simulink model "cbf_with_lead_accel_est"  (R2021a)
settings: Solver=FixedStepAuto  StartTime=0.0  StopTime=inf  FixedStep=0.05  RelTol=1e-3
undefined symbols (not defined in the file): Angular, Linear
libraries: robotlib x18
settings Model: Creator=ivory  LastModifiedBy=vanderbilt
settings SolverCC: AlgebraicLoopSolver=TrustRegion
settings OptimizationCC: EnhancedBackFolding=on  PassReuseOutputArgsAs=Individual arguments  ZeroExternalMemoryAtStartup=off  ZeroInternalMemoryAtStartup=off  MaxStackSize=64  OptimizeBlockOrder=speed  DifferentSizesBufferReuse=on  OptimizationCustomize=off  EfficientTunableParamExpr=on
settings DebuggingCC: ParameterTunabilityLossMsg=error  SFMachineParentedDataDiag=warning
settings HardwareCC: ProdBitPerPointer=32  ProdBitPerSizeT=32  ProdBitPerPtrDiffT=32  ProdLargestAtomicFloat=None  ProdIntDivRoundTo=Undefined  ProdEndianess=Unspecified  ProdWordSize=32  ProdHWDeviceType=Generic->Unspecified (assume 32-bit Generic)
settings SFSimCC: MATLABDynamicMemAlloc=off  SimTargetLang=C++
settings RTWCC: SystemTargetFile=ert.tlc  HardwareBoard=Robot Operating System (ROS)  TLCOptions="-aInlineSetEventsForThisBaseRateFcn=TLC_FALSE -aSuppressMultiTaskScheduler=TLC_FALSE  -aRateBasedStepFcn=0"  TemplateMakefile=ert_default_tmf  GenerateReport=on  Toolchain=Catkin  IncludeHyperlinkInReport=on  LaunchReport=on  TargetLang=C++  GenerateTraceInfo=on  GenerateTraceReport=on  GenerateTraceReportSl=on  GenerateTraceReportSf=on  GenerateTraceReportEml=on
settings CodeAppCC: ForceParamTrailComments=on  IgnoreCustomStorageClasses=off  OperatorAnnotations=on  SimulinkDataObjDesc=on  SFDataObjDesc=on  InsertBlockDesc=on
settings ERTTargetCC: SupportContinuousTime=on  SupportVariableSizeSignals=on

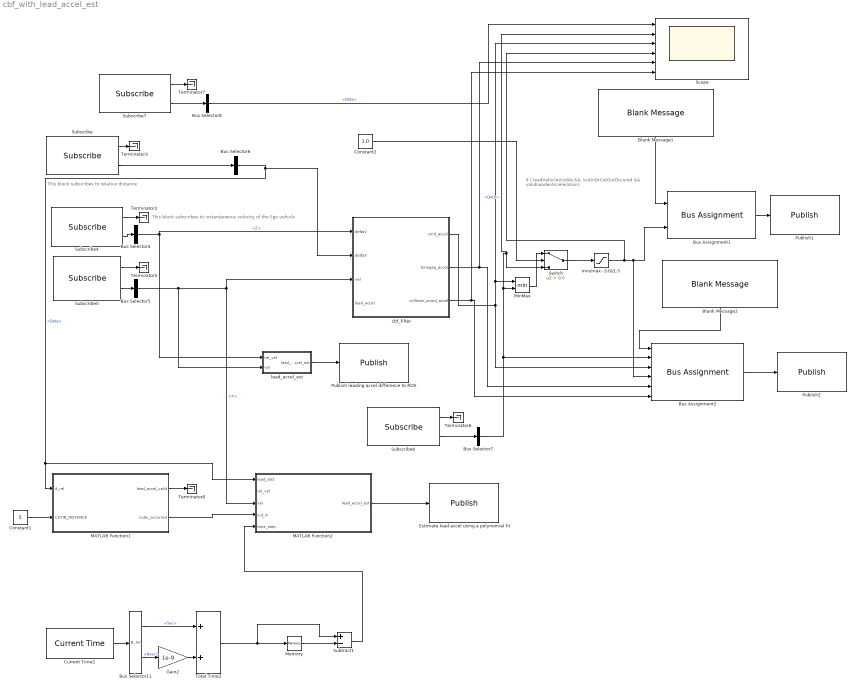
== system cbf_with_lead_accel_est ==
  note: if ( leadVehicleVisible && !cutInOrCutOutOccured && validLeaderAcceleration)
  note: This block subscribes
      | to relative distance
  note: This block subscribes to
      | instantaneous velocity of the Ego vehicle
  Blank Message1 : robotlib/Blank Message  messageClass=Message  entityType=std_msgs/Float64  messageType=std_msgs/Float64  SampleTime=inf  legacyBusStruct=off
  Blank Message2 : robotlib/Blank Message  messageClass=Message  entityType=geometry_msgs/Twist  messageType=geometry_msgs/Twist  SampleTime=inf  legacyBusStruct=off
  Bus Assignment1 : BusAssignment  AssignedSignals=Data
  Bus Assignment2 : BusAssignment  AssignedSignals=Linear.X,Linear.Y,Linear.Z,Angular.Y,Angular.Z
  Bus Selector11 : BusSelector  OutputSignals=Sec,Nsec
  Bus Selector4 : BusSelector  OutputSignals=Linear.Z
  Bus Selector5 : BusSelector  OutputSignals=Linear.X
  Bus Selector6 : BusSelector  OutputSignals=Data
  Bus Selector7 : BusSelector  OutputSignals=Data
  Bus Selector8 : BusSelector  OutputSignals=Data
  Constant1 : Constant  Value=5
  Constant2 : Constant  Value=1.0
  Current Time2 : robotlib/Current Time  OutputFormat=bus  SampleTime=-1  ModelName=micromodel
      settings: SourceProductBaseCode=RR
  Estimate lead accel using a polynomial fit : robotlib/Publish  topicSource=Specify your own  topic=/lead_accel_est/polynomial_est  messageType=std_msgs/Float64  legacyBusStruct=off  messageQueueLength=1
  Gain2 : Gain  Gain=1e-9
  MATLAB Function1 : MATLAB Function  TreatAsAtomicUnit=on
  MATLAB Function2 : MATLAB Function  TreatAsAtomicUnit=on
  Memory : Memory
  MinMax : MinMax  Inputs=2
  Publish leading accel difference to ROS : robotlib/Publish  topicSource=Specify your own  topic=/lead_accel_est/finite_diff  messageType=std_msgs/Float64  legacyBusStruct=off  messageQueueLength=1
  Publish1 : robotlib/Publish  topicSource=Specify your own  topic=cmd_accel  messageType=std_msgs/Float64  legacyBusStruct=off  messageQueueLength=1
  Publish2 : robotlib/Publish  topicSource=Specify your own  topic=/cbf/cbf_debug  messageType=geometry_msgs/Twist  legacyBusStruct=off  messageQueueLength=1
  Scope : Scope  NumInputPorts=6
  Subscribe : robotlib/Subscribe  topicSource=Specify your own  topic=lead_dist  messageType=std_msgs/Float64  SampleTime=-1  legacyBusStruct=off  messageQueueLength=1
  Subscribe4 : robotlib/Subscribe  topicSource=Specify your own  topic=rel_vel  messageType=geometry_msgs/Twist  SampleTime=-1  legacyBusStruct=off  messageQueueLength=1
  Subscribe5 : robotlib/Subscribe  topicSource=Specify your own  topic=vel  messageType=geometry_msgs/Twist  SampleTime=-1  legacyBusStruct=off  messageQueueLength=1
  Subscribe6 : robotlib/Subscribe  topicSource=Specify your own  topic=cmd_accel_pre  messageType=std_msgs/Float64  SampleTime=-1  legacyBusStruct=off  messageQueueLength=1
  Subscribe7 : robotlib/Subscribe  topicSource=Specify your own  topic=/car/hud/mini_car_enable  messageType=std_msgs/Bool  SampleTime=-1  legacyBusStruct=off  messageQueueLength=1
  Subtract1 : Sum  Inputs=+-
  Switch : Switch  Criteria=u2 > Threshold  Threshold=0.5
  Terminator{2..3,5..8} (6 alike) : Terminator
  Total Time2 : Sum
  cbf_filter : Subsystem
  lead_accel_est : Subsystem
  min/max -3.0//1.5 : Saturate  UpperLimit=1.5  LowerLimit=-3.0
  wires:
  Subscribe4/1 -> Terminator2/1
  Bus Selector4/1 -> lead_accel_est/1(rel_vel), cbf_filter/1(deltaV)  "<Z>"
  Subscribe5/2 -> Bus Selector5/1
  Subscribe4/2 -> Bus Selector4/1
  Bus Selector5/1 -> lead_accel_est/2(vel), MATLAB Function2/3(vel), cbf_filter/3(vel)  "<X>"
  Bus Assignment1/1 -> Publish1/1
  Blank Message1/1 -> Bus Assignment1/1
  Subscribe5/1 -> Terminator5/1
  Subscribe/1 -> Terminator3/1
  Subscribe/2 -> Bus Selector6/1
  Bus Selector6/1 -> MATLAB Function2/1(lead_dist), MATLAB Function1/1(d_rel), cbf_filter/2(deltaX)  "<Data>"
  Subscribe6/2 -> Bus Selector7/1
  Bus Selector7/1 -> Bus Assignment2/2, MinMax/2, Switch/3, Scope/2  "<Data>"
  Subscribe6/1 -> Terminator6/1
  Subscribe7/2 -> Bus Selector8/1
  Subscribe7/1 -> Terminator7/1
  Bus Selector8/1 -> Scope/1  "<Data>"
  Constant1/1 -> MATLAB Function1/2(CUTIN_DISTANCE)
  cbf_filter/1(cmd_accel) -> Scope/3, MinMax/1, Bus Assignment2/3
  MinMax/1 -> Switch/1
  min/max -3.0//1.5/1 -> Scope/4, Bus Assignment2/4, Bus Assignment1/2
  Blank Message2/1 -> Bus Assignment2/1
  Bus Assignment2/1 -> Publish2/1
  cbf_filter/2(timegap_accel) -> Scope/5, Bus Assignment2/5
  cbf_filter/3(collision_avoid_accel) -> Scope/6, Bus Assignment2/6
  MATLAB Function1/1(lead_accel_valid) -> Terminator8/1
  MATLAB Function1/2(cutin_occurred) -> MATLAB Function2/4(cut_in)
  Switch/1 -> min/max -3.0//1.5/1
  Constant2/1 -> Switch/2
  lead_accel_est/1(lead_accel_est) -> Publish leading accel difference to ROS/1
  MATLAB Function2/1(lead_accel_est) -> Estimate lead accel using a polynomial fit/1
  Gain2/1 -> Total Time2/2
  Bus Selector11/2 -> Gain2/1  "<Nsec>"
  Bus Selector11/1 -> Total Time2/1  "<Sec>"
  Memory/1 -> Subtract1/2
  Current Time2/1 -> Bus Selector11/1
  Total Time2/1 -> Subtract1/1, Memory/1
  Subtract1/1 -> MATLAB Function2/5(time_step)

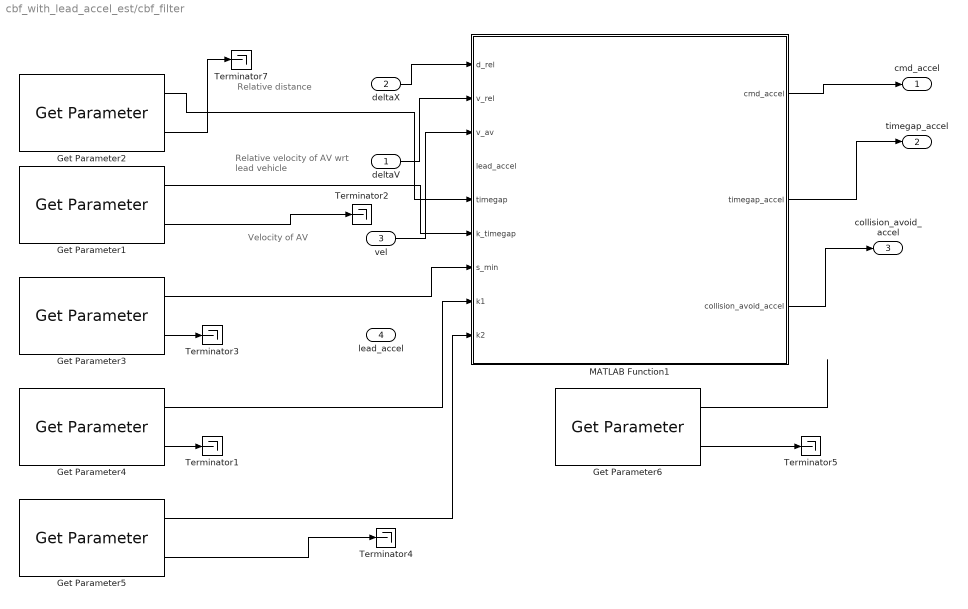
== system cbf_with_lead_accel_est/cbf_filter ==
  note: Velocity of AV
  note: Relative velocity of
      | AV wrt lead vehicle
  note: Relative distance
  deltaV : Inport
  deltaX : Inport  Port=2
  vel : Inport  Port=3
  lead_accel : Inport  Port=4
  Get Parameter1 : robotlib/Get Parameter  ParameterSource=Specify your own  ParameterName=k_timegap  ParameterType=double  ParameterMaxArrayLength=16  ParameterInitialValue=0.1  SampleTime=-1  ShowErrorCodeOutput=on  ModelName=cbf_with_lead_accel_est  BlockId=ParamGet_cbf_with_lead_accel_est_447
      settings: SourceProductBaseCode=RR
  Get Parameter2 : robotlib/Get Parameter  ParameterSource=Specify your own  ParameterName=timegap  ParameterType=double  ParameterMaxArrayLength=16  ParameterInitialValue=2.0  SampleTime=-1  ShowErrorCodeOutput=on  ModelName=cbf_with_lead_accel_est  BlockId=ParamGet_cbf_with_lead_accel_est_448
      settings: SourceProductBaseCode=RR
  Get Parameter3 : robotlib/Get Parameter  ParameterSource=Specify your own  ParameterName=s_min  ParameterType=double  ParameterMaxArrayLength=16  ParameterInitialValue=15.0  SampleTime=-1  ShowErrorCodeOutput=on  ModelName=cbf_with_lead_accel_est  BlockId=ParamGet_cbf_with_lead_accel_est_449
      settings: SourceProductBaseCode=RR
  Get Parameter4 : robotlib/Get Parameter  ParameterSource=Specify your own  ParameterName=k1  ParameterType=double  ParameterMaxArrayLength=16  ParameterInitialValue=0.5  SampleTime=-1  ShowErrorCodeOutput=on  ModelName=cbf_with_lead_accel_est  BlockId=ParamGet_cbf_with_lead_accel_est_450
      settings: SourceProductBaseCode=RR
  Get Parameter5 : robotlib/Get Parameter  ParameterSource=Specify your own  ParameterName=k2  ParameterType=double  ParameterMaxArrayLength=16  ParameterInitialValue=0.5  SampleTime=-1  ShowErrorCodeOutput=on  ModelName=cbf_with_lead_accel_est  BlockId=ParamGet_cbf_with_lead_accel_est_463
      settings: SourceProductBaseCode=RR
  Get Parameter6 : robotlib/Get Parameter  ParameterSource=Specify your own  ParameterName=w3  ParameterType=double  ParameterMaxArrayLength=16  ParameterInitialValue=6.0  SampleTime=-1  ShowErrorCodeOutput=on  ModelName=cbf_with_lead_accel_est  BlockId=ParamGet_cbf_with_lead_accel_est_465
      settings: SourceProductBaseCode=RR
  MATLAB Function1 : MATLAB Function  TreatAsAtomicUnit=on
  Terminator{1..5,7} (6 alike) : Terminator
  cmd_accel : Outport
  timegap_accel : Outport  Port=2
  collision_avoid_accel : Outport  Port=3
  wires:
  Get Parameter4/1 -> MATLAB Function1/8(k1)
  Get Parameter4/2 -> Terminator1/1
  Get Parameter2/1 -> MATLAB Function1/5(timegap)
  Get Parameter2/2 -> Terminator7/1
  Get Parameter3/2 -> Terminator3/1
  Get Parameter1/1 -> MATLAB Function1/6(k_timegap)
  Get Parameter1/2 -> Terminator2/1
  Get Parameter3/1 -> MATLAB Function1/7(s_min)
  MATLAB Function1/2(timegap_accel) -> timegap_accel/1
  MATLAB Function1/1(cmd_accel) -> cmd_accel/1
  vel/1 -> MATLAB Function1/3(v_av)
  deltaV/1 -> MATLAB Function1/2(v_rel)
  deltaX/1 -> MATLAB Function1/1(d_rel)
  Get Parameter5/2 -> Terminator4/1
  Get Parameter5/1 -> MATLAB Function1/9(k2)
  Get Parameter6/1 -> ?
  Get Parameter6/2 -> Terminator5/1
  MATLAB Function1/3(collision_avoid_accel) -> collision_avoid_accel/1

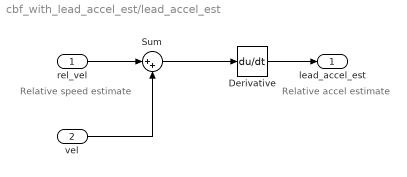
== system cbf_with_lead_accel_est/lead_accel_est ==
  note: Relative speed estimate
  note: Relative accel estimate
  rel_vel : Inport
  vel : Inport  Port=2
  Derivative : Derivative
  Sum : Sum  Inputs=|++
  lead_accel_est : Outport
  wires:
  rel_vel/1 -> Sum/1
  Derivative/1 -> lead_accel_est/1
  vel/1 -> Sum/2
  Sum/1 -> Derivative/1

== matlab function cbf_with_lead_accel_est/MATLAB Function2 ==
  data: lead_accel_est output; lead_dist input; rel_vel input; vel input; cut_in input; time_step input
function lead_accel_est = fcn(lead_dist,rel_vel,vel,cut_in,time_step)
%#codegen

%% Make persistent variables that we'll need:


persistent num_samples_current
persistent lead_vel_history

if cut_in
    rel_vel_history = zeros(num_samples_current,1);
else
    lead_vel_est = vel + rel_vel;
    rel_vel_history
    
end


if isempty(time_avg_target)
    t_length= 1;
    time_avg_target = zeros(1, 1280);% Data Rate = 20 Hz, To consider 64 seconds, 20*64 data points are required
    time_avg_target(1280)= lead_vel;
else
    time_avg_target = [time_avg_target(2:end),lead_vel];
    if(t_length < 1280)
        t_length= t_length + 1;
    end
end



persistent relative_distance_prev;
if isempty(relative_distance_prev)
    relative_distance_prev=d_rel;
end

cutin_occurred = 1;
lead_accel_valid=1;

if( abs( relative_distance_prev - d_rel ) > CUTIN_DISTANCE )
    cutin_occurred = 1;
else
    cutin_occurred = 0;
end

relative_distance_prev = d_rel;



end

== matlab function cbf_with_lead_accel_est/cbf_filter/MATLAB Function1 ==
  data: cmd_accel output; d_rel input; v_rel input; v_av input; lead_accel input; timegap input; timegap_accel output; collision_avoid_accel output; k_timegap input; s_min input; k1 input; k2 input
function [cmd_accel, timegap_accel, collision_avoid_accel]= fcn(d_rel,v_rel,v_av,lead_accel, timegap,k_timegap,s_min,k1,k2)
%#codegen

% from the timegap filter function
% maybe make this gain a parameter later
% k = 0.1;
k = k_timegap;
%t_min = 2.0;
t_min = timegap;
timegap_accel = (1/t_min)*v_rel + (k/t_min)*(d_rel - t_min*v_av);

% from collision-avoid filter function
% a potential parameter - read into the fcn now
% s_min = 15.0;
% a potential parameter - read into the fcn now
% k1 = 0.5;
% a potential parameter - read into the fcn now
% k2 = 0.5;
%a_max = a_l + (k1+k2)*(delta_v) + (k1*k2)*(s-s_min);


% simplification TODO this is maybe dangerous so need to confirm
a_l = 0;
collision_avoid_accel = a_l + (k1+k2)*(v_rel) + (k1*k2)*(d_rel-s_min);

cmd_accel = min(timegap_accel,collision_avoid_accel);

== matlab function cbf_with_lead_accel_est/MATLAB Function1 ==
  data: lead_accel_valid output; d_rel input; CUTIN_DISTANCE input; cutin_occurred output
function [lead_accel_valid, cutin_occurred]= fcn(d_rel,CUTIN_DISTANCE)
%#codegen

persistent relative_distance_prev;
if isempty(relative_distance_prev)
    relative_distance_prev=d_rel;
end

cutin_occurred = 1;
lead_accel_valid=1;

if( abs( relative_distance_prev - d_rel ) > CUTIN_DISTANCE )
    cutin_occurred = 1;
else
    cutin_occurred = 0;
end

relative_distance_prev = d_rel;
